simulink library "tqr"  (R2021b)
settings: Solver=VariableStepAuto  StartTime=0.0  StopTime=10.0  RelTol=1e-3
undefined symbols (not defined in the file or in its folder): ATQR_AltRDCActiveFEDUInc_X_pct, ATQR_AltRDCActiveFEDUInc_Y_enum, ATQR_AltRDCActiveFEDUTs_X_pct, ATQR_AltRDCActiveFEDUTs_Y_enum, ATQR_AltRDCActiveREDUInc_X_pct, ATQR_AltRDCActiveREDUInc_Y_enum, ATQR_AltRDCActiveREDUTs_X_pct, ATQR_AltRDCActiveREDUTs_Y_enum, ATQR_CreepFEDUTqIncSR_X_rpm, ATQR_CreepFEDUTqIncSR_Y_Nm, ATQR_CreepFEDUTs_X_rpm, ATQR_CreepFEDUTs_Y_Nm, ATQR_ECO2TqFrIncGain_X_Nm, ATQR_ECO2TqFrIncGain_Y_pct, ATQR_ECO2TqRrIncGain_X_Nm, ATQR_ECO2TqRrIncGain_Y_pct, ATQR_EcoTqFrIncGain_X_Nm, ATQR_EcoTqFrIncGain_Y_pct, ATQR_EcoTqRrIncGain_X_Nm, ATQR_EcoTqRrIncGain_Y_pct, ATQR_EL1FEDUTqDecSR_Y_Nm, ATQR_EL1FEDUTqIncSR_X_rpm, ATQR_EL1FEDUTqIncSR_Y_pct, ATQR_EL1FEDUTs_X_rpm, ATQR_EL1FEDUTs_Y_Nm, ATQR_EL1REDUTqDecSR_Y_Nm, ATQR_EL1REDUTs_Y_Nm, ATQR_FEDUEL1RegenTs_X_rpm, ATQR_FEDUTIPOutTs_X_rpm, ATQR_FrNegRateLimitIncN_X_rpm, ATQR_FrNegRateLimitIncN_Y_Nm, ATQR_FrPosRateLimitIncN_X_rpm, ATQR_FrPosRateLimitIncN_Y_Nm, ATQR_FShaftSpdTqLimCoe_X_rpm, ATQR_FTimerTqLimCoe_X_s, ATQR_FTqZeroTransUpBoundN_X_rpm, ATQR_NL1FEDUTqDecSR_Y_Nm, ATQR_NL1FEDUTqIncSR_X_rpm, ATQR_NL1FEDUTqIncSR_Y_pct, ATQR_NL1FEDUTs_X_rpm, ATQR_NL1FEDUTs_Y_Nm, ATQR_NL1REDUTqDecSR_Y_Nm, ATQR_NL1REDUTs_Y_Nm, ATQR_NL2TqFrIncGain_X_Nm, ATQR_NL2TqFrIncGain_Y_pct, ATQR_NL2TqRrIncGain_X_Nm, ATQR_NL2TqRrIncGain_Y_pct, ATQR_NormalTqFrIncGain_X_Nm, ATQR_NormalTqFrIncGain_Y_pct, ATQR_NormalTqRrIncGain_X_Nm, ATQR_NormalTqRrIncGain_Y_pct, ATQR_RrNegRateLimitIncN_X_rpm, ATQR_RrNegRateLimitIncN_Y_Nm, ATQR_RrPosRateLimitIncN_X_rpm, ATQR_RrPosRateLimitIncN_Y_Nm, ATQR_RShaftSpdTqLimCoe_X_rpm, ATQR_RTimerTqLimCoe_X_s, ATQR_SL1FEDUTqDecSR_Y_Nm, ATQR_SL1FEDUTqIncSR_X_rpm, ATQR_SL1FEDUTqIncSR_Y_pct ... (+344)
libraries: hcu_lib x23, simulink x17, $bdroot x3
(part 9 of 12)

== system tqr/TQR/Determine Torque Request/TorqueArbitrament/TorqueSmooth/Rear wheel rate limit determination/VTQR_ECOREDURateLimitInc_Nm ==
  VDHP_ActAPSPosn_pct : Inport
  VTQD_TqTargetShaftSpd_rpm : Inport  Port=2
  VTQD_RegenMode_enum : Inport  Port=3
  VTQR_REDUWhlTqReqSmoothDelay_Nm : Inport  Port=4
  Action Port : ActionPort
  Constant : Constant  Value=ENUM_REGENLEVEL_LV1
  Constant1 : Constant  Value=ENUM_REGENLEVEL_LV2
  Constant2 : Constant  Value=ENUM_REGENLEVEL_LV3
  Constant3 : Constant  Value=ENUM_REGENLEVEL_LV4
  Constant4 : Constant  Value=ENUM_REGENLEVEL_LV5
  Constant5 : Constant  Value=ENUM_REGENLEVEL_OPD
  Constant6 : Constant  Value=KTQR_EnEcoRrIncGain_enum
  Constant7 : Constant  Value=ONE_FLOAT
  Equal{,1..5} (6 alike) : RelationalOperator  Operator===  OutDataTypeStr=boolean  RndMeth=Simplest
  If : If  NumInputs=6  IfExpression=u1~= 0  ElseIfExpressions=u2 ~= 0, u3 ~= 0,u4 ~= 0,u5~=0,u6~=0
  Invalid : Subsystem  TreatAsAtomicUnit=on
  LV1 : Subsystem  TreatAsAtomicUnit=on
  LV2 : Subsystem  TreatAsAtomicUnit=on
  LV3 : Subsystem  TreatAsAtomicUnit=on
  LV4 : Subsystem  TreatAsAtomicUnit=on
  LV5 : Subsystem  TreatAsAtomicUnit=on
  MTQR_ECO2TqRrIncGain_Z_c : Lookup_n-D  BreakpointsForDimension1=ATQR_ECO2TqRrIncGain_Y_pct  BreakpointsForDimension2=ATQR_ECO2TqRrIncGain_X_Nm  Table=MTQR_ECO2TqRrIncGain_Z_c  ExtrapMethod=Clip  InternalRulePriority=Speed  RndMeth=Simplest  InputSameDT=on
      settings: InputPortMap=u0,u1
  MTQR_ECO3TqRrIncGain_Z_c : Lookup_n-D  BreakpointsForDimension1=ATQR_ECO2TqRrIncGain_Y_pct  BreakpointsForDimension2=ATQR_ECO2TqRrIncGain_X_Nm  Table=MTQR_ECO3TqRrIncGain_Z_c  ExtrapMethod=Clip  InternalRulePriority=Speed  RndMeth=Simplest  InputSameDT=on
      settings: InputPortMap=u0,u1
  MTQR_ECO4TqRrIncGain_Z_c : Lookup_n-D  BreakpointsForDimension1=ATQR_ECO2TqRrIncGain_Y_pct  BreakpointsForDimension2=ATQR_ECO2TqRrIncGain_X_Nm  Table=MTQR_ECO4TqRrIncGain_Z_c  ExtrapMethod=Clip  InternalRulePriority=Speed  RndMeth=Simplest  InputSameDT=on
      settings: InputPortMap=u0,u1
  MTQR_ECO5TqRrIncGain_Z_c : Lookup_n-D  BreakpointsForDimension1=ATQR_ECO2TqRrIncGain_Y_pct  BreakpointsForDimension2=ATQR_ECO2TqRrIncGain_X_Nm  Table=MTQR_ECO5TqRrIncGain_Z_c  ExtrapMethod=Clip  InternalRulePriority=Speed  RndMeth=Simplest  InputSameDT=on
      settings: InputPortMap=u0,u1
  MTQR_ECOOPDTqRrIncGain_Z_c : Lookup_n-D  BreakpointsForDimension1=ATQR_ECO2TqRrIncGain_Y_pct  BreakpointsForDimension2=ATQR_ECO2TqRrIncGain_X_Nm  Table=MTQR_ECOOPDTqRrIncGain_Z_c  ExtrapMethod=Clip  InternalRulePriority=Speed  RndMeth=Simplest  InputSameDT=on
      settings: InputPortMap=u0,u1
  MTQR_EcoTqRrIncGain_Z_c : Lookup_n-D  BreakpointsForDimension1=ATQR_EcoTqRrIncGain_Y_pct  BreakpointsForDimension2=ATQR_EcoTqRrIncGain_X_Nm  Table=MTQR_EcoTqRrIncGain_Z_c  ExtrapMethod=Clip  InternalRulePriority=Speed  RndMeth=Simplest  InputSameDT=on
      settings: InputPortMap=u0,u1
  Merge : Merge  Inputs=7
  OPD : Subsystem  TreatAsAtomicUnit=on
  Relational Operator : RelationalOperator  OutDataTypeStr=boolean  RndMeth=Simplest
  Switch : Switch  Criteria=u2 > Threshold
  VTQR_ECOREDURateLimitInc_Nm : Outport
  wires:
  [VDHP_ActAPSPosn_pct] -> MTQR_ECOOPDTqRrIncGain_Z_c/1
  [VTQR_REDUWhlTqReqSmoothDelay_Nm] -> MTQR_ECOOPDTqRrIncGain_Z_c/2
  [VDHP_ActAPSPosn_pct] -> MTQR_ECO5TqRrIncGain_Z_c/1
  [VTQR_REDUWhlTqReqSmoothDelay_Nm] -> MTQR_ECO5TqRrIncGain_Z_c/2
  [VTQR_REDUWhlTqReqSmoothDelay_Nm] -> MTQR_ECO4TqRrIncGain_Z_c/2
  [VDHP_ActAPSPosn_pct] -> MTQR_ECO4TqRrIncGain_Z_c/1
  [VTQR_REDUWhlTqReqSmoothDelay_Nm] -> MTQR_ECO3TqRrIncGain_Z_c/2
  [VDHP_ActAPSPosn_pct] -> MTQR_ECO3TqRrIncGain_Z_c/1
  [VTQR_REDUWhlTqReqSmoothDelay_Nm] -> MTQR_ECO2TqRrIncGain_Z_c/2
  [VDHP_ActAPSPosn_pct] -> MTQR_ECO2TqRrIncGain_Z_c/1
  If/7 -> Invalid/Action
  If/6 -> OPD/Action
  [VTQR_ECOOPDTqRrIncGain_c] -> OPD/4(VTQR_ECOOPDTqRrIncGain_c)
  If/5 -> LV5/Action
  [VTQR_ECO5TqRrIncGain_c] -> LV5/4(VTQR_ECO5TqRrIncGain_c)
  If/4 -> LV4/Action
  [VTQR_ECO4TqRrIncGain_c] -> LV4/4(VTQR_ECO4TqRrIncGain_c)
  If/3 -> LV3/Action
  [VTQR_ECO3TqRrIncGain_c] -> LV3/4(VTQR_ECO3TqRrIncGain_c)
  If/2 -> LV2/Action
  [VTQR_ECO2TqRrIncGain_c] -> LV2/4(VTQR_ECO2TqRrIncGain_c)
  If/1 -> LV1/Action
  MTQR_ECO5TqRrIncGain_Z_c/1 -> [VTQR_ECO5TqRrIncGain_c]  "VTQR_ECO5TqRrIncGain_c"
  MTQR_ECO2TqRrIncGain_Z_c/1 -> [VTQR_ECO2TqRrIncGain_c]  "VTQR_ECO2TqRrIncGain_c"
  MTQR_ECOOPDTqRrIncGain_Z_c/1 -> [VTQR_ECOOPDTqRrIncGain_c]  "VTQR_ECOOPDTqRrIncGain_c"
  MTQR_ECO3TqRrIncGain_Z_c/1 -> [VTQR_ECO3TqRrIncGain_c]  "VTQR_ECO3TqRrIncGain_c"
  MTQR_ECO4TqRrIncGain_Z_c/1 -> [VTQR_ECO4TqRrIncGain_c]  "VTQR_ECO4TqRrIncGain_c"
  Switch/1 -> [VTQR_EcoTqRrIncGain_c]  "VTQR_EcoTqRrIncGain_c"
  MTQR_EcoTqRrIncGain_Z_c/1 -> Switch/1
  [VTQD_RegenMode_enum] -> Relational Operator/1
  Constant6/1 -> Relational Operator/2
  Constant7/1 -> Switch/3
  Relational Operator/1 -> Switch/2
  [VTQR_EcoTqRrIncGain_c] -> OPD/3(VTQR_EcoTqRrIncGain_c)
  [VTQR_EcoTqRrIncGain_c] -> LV5/3(VTQR_EcoTqRrIncGain_c)
  [VTQR_EcoTqRrIncGain_c] -> LV4/3(VTQR_EcoTqRrIncGain_c)
  [VTQR_EcoTqRrIncGain_c] -> LV3/3(VTQR_EcoTqRrIncGain_c)
  [VTQR_EcoTqRrIncGain_c] -> LV2/3(VTQR_EcoTqRrIncGain_c)
  [VTQR_EcoTqRrIncGain_c] -> LV1/3(VTQR_EcoTqRrIncGain_c)
  VTQR_REDUWhlTqReqSmoothDelay_Nm/1 -> [VTQR_REDUWhlTqReqSmoothDelay_Nm]
  [VDHP_ActAPSPosn_pct] -> MTQR_EcoTqRrIncGain_Z_c/1
  [VTQR_REDUWhlTqReqSmoothDelay_Nm] -> MTQR_EcoTqRrIncGain_Z_c/2
  Invalid/1(VTQR_EL1REDUTqIncSR_Nm) -> Merge/7
  [VTQD_TqTargetShaftSpd_rpm] -> Invalid/2(VTQD_TqTargetShaftSpd_rpm)
  [VDHP_ActAPSPosn_pct] -> Invalid/1(VDHP_ActAPSPosn_pct)
  VTQD_RegenMode_enum/1 -> [VTQD_RegenMode_enum]
  VTQD_TqTargetShaftSpd_rpm/1 -> [VTQD_TqTargetShaftSpd_rpm]
  VDHP_ActAPSPosn_pct/1 -> [VDHP_ActAPSPosn_pct]
  Merge/1 -> VTQR_ECOREDURateLimitInc_Nm/1  "VTQR_ECOREDURateLimitInc_Nm"
  Constant2/1 -> Equal2/2
  [VDHP_ActAPSPosn_pct] -> LV1/1(VDHP_ActAPSPosn_pct)
  [VTQD_TqTargetShaftSpd_rpm] -> LV3/2(VTQD_TqTargetShaftSpd_rpm)
  LV4/1(VTQR_EL4REDUTqIncSR_Nm) -> Merge/4
  Equal3/1 -> If/4
  [VTQD_RegenMode_enum] -> Equal1/1
  LV5/1(VTQR_EL5REDUTqIncSR_Nm) -> Merge/5
  LV3/1(VTQR_EL3REDUTqIncSR_Nm) -> Merge/3
  [VTQD_RegenMode_enum] -> Equal3/1
  Equal1/1 -> If/2
  Equal4/1 -> If/5
  [VTQD_RegenMode_enum] -> Equal/1
  LV1/1(VTQR_EL1REDUTqIncSR_Nm) -> Merge/1
  Constant1/1 -> Equal1/2
  Equal/1 -> If/1
  [VTQD_TqTargetShaftSpd_rpm] -> LV5/2(VTQD_TqTargetShaftSpd_rpm)
  [VDHP_ActAPSPosn_pct] -> LV4/1(VDHP_ActAPSPosn_pct)
  Constant5/1 -> Equal5/2
  [VDHP_ActAPSPosn_pct] -> LV3/1(VDHP_ActAPSPosn_pct)
  [VTQD_TqTargetShaftSpd_rpm] -> LV4/2(VTQD_TqTargetShaftSpd_rpm)
  [VTQD_TqTargetShaftSpd_rpm] -> OPD/2(VTQD_TqTargetShaftSpd_rpm)
  [VDHP_ActAPSPosn_pct] -> LV5/1(VDHP_ActAPSPosn_pct)
  [VTQD_TqTargetShaftSpd_rpm] -> LV1/2(VTQD_TqTargetShaftSpd_rpm)
  [VTQD_RegenMode_enum] -> Equal2/1
  [VDHP_ActAPSPosn_pct] -> OPD/1(VDHP_ActAPSPosn_pct)
  [VTQD_RegenMode_enum] -> Equal5/1
  LV2/1(VTQR_EL2REDUTqIncSR_Nm) -> Merge/2
  [VDHP_ActAPSPosn_pct] -> LV2/1(VDHP_ActAPSPosn_pct)
  [VTQD_RegenMode_enum] -> Equal4/1
  OPD/1(VTQR_EOPDREDUTqIncSR_Nm) -> Merge/6
  Equal5/1 -> If/6
  Constant/1 -> Equal/2
  Constant4/1 -> Equal4/2
  Equal2/1 -> If/3
  Constant3/1 -> Equal3/2
  [VTQD_TqTargetShaftSpd_rpm] -> LV2/2(VTQD_TqTargetShaftSpd_rpm)

== system tqr/TQR/Determine Torque Request/TorqueArbitrament/TorqueSmooth/Rear wheel rate limit determination/VTQR_ESCAPEREDURateLimitDec_Nm ==
  VTQR_REDUWhlTqReqSmoothDelay_Nm : Inport
  VTQD_RrShaftSpd_rpm : Inport  Port=2
  Action Port : ActionPort
  MTQR_ESCAPEREDUTqDecSR_Z_Nm : Lookup_n-D  BreakpointsForDimension1=ATQR_NL1REDUTqDecSR_Y_Nm  BreakpointsForDimension2=ATQR_NL1FEDUTqIncSR_X_rpm  Table=MTQR_ESCAPEREDUTqDecSR_Z_Nm  InternalRulePriority=Speed  RndMeth=Simplest  InputSameDT=on
      settings: InputPortMap=u0,u1
  VTQR_ESCAPEREDURateLimitDec_Nm : Outport
  wires:
  MTQR_ESCAPEREDUTqDecSR_Z_Nm/1 -> VTQR_ESCAPEREDURateLimitDec_Nm/1
  VTQR_REDUWhlTqReqSmoothDelay_Nm/1 -> MTQR_ESCAPEREDUTqDecSR_Z_Nm/1
  VTQD_RrShaftSpd_rpm/1 -> MTQR_ESCAPEREDUTqDecSR_Z_Nm/2

== system tqr/TQR/Determine Torque Request/TorqueArbitrament/TorqueSmooth/Rear wheel rate limit determination/VTQR_ESCAPEREDURateLimitInc_Nm ==
  VDHP_ActAPSPosn_pct : Inport
  VTQD_RrShaftSpd_rpm : Inport  Port=2
  Action Port : ActionPort
  MTQR_ESCAPEREDUTqIncSR_Z_Nm : Lookup_n-D  BreakpointsForDimension1=ATQR_NL1FEDUTqIncSR_Y_pct  BreakpointsForDimension2=ATQR_NL1FEDUTqIncSR_X_rpm  Table=MTQR_ESCAPEREDUTqIncSR_Z_Nm  InternalRulePriority=Speed  RndMeth=Simplest  InputSameDT=on
      settings: InputPortMap=u0,u1
  VTQR_ESCAPEREDURateLimitInc_Nm : Outport
  wires:
  VDHP_ActAPSPosn_pct/1 -> MTQR_ESCAPEREDUTqIncSR_Z_Nm/1
  VTQD_RrShaftSpd_rpm/1 -> MTQR_ESCAPEREDUTqIncSR_Z_Nm/2
  MTQR_ESCAPEREDUTqIncSR_Z_Nm/1 -> VTQR_ESCAPEREDURateLimitInc_Nm/1

== system tqr/TQR/Determine Torque Request/TorqueArbitrament/TorqueSmooth/Rear wheel rate limit determination/VTQR_LHMREDURateLimitDec_Nm ==
  VTQR_REDUWhlTqReqSmooth_Nm : Inport
  VTQD_TqTargetShaftSpd_rpm : Inport  Port=2
  Action Port : ActionPort
  MTQR_LHMREDUTqDecSR_Z_Nm : Lookup_n-D  BreakpointsForDimension1=ATQR_NL1REDUTqDecSR_Y_Nm  BreakpointsForDimension2=ATQR_NL1FEDUTqIncSR_X_rpm  Table=MTQR_LHMREDUTqDecSR_Z_Nm  ExtrapMethod=Clip  InternalRulePriority=Speed  RndMeth=Simplest  InputSameDT=on
      settings: InputPortMap=u0,u1
  VTQR_LHMREDURateLimitDec_Nm : Outport
  wires:
  MTQR_LHMREDUTqDecSR_Z_Nm/1 -> VTQR_LHMREDURateLimitDec_Nm/1  "VTQR_LHMREDURateLimitDec_Nm"
  VTQD_TqTargetShaftSpd_rpm/1 -> MTQR_LHMREDUTqDecSR_Z_Nm/2
  VTQR_REDUWhlTqReqSmooth_Nm/1 -> MTQR_LHMREDUTqDecSR_Z_Nm/1

== system tqr/TQR/Determine Torque Request/TorqueArbitrament/TorqueSmooth/Rear wheel rate limit determination/VTQR_LHMREDURateLimitInc_Nm ==
  VDHP_ActAPSPosn_pct : Inport
  VTQD_TqTargetShaftSpd_rpm : Inport  Port=2
  Action Port : ActionPort
  MTQR_LHMREDUTqIncSR_Z_Nm : Lookup_n-D  BreakpointsForDimension1=ATQR_NL1FEDUTqIncSR_Y_pct  BreakpointsForDimension2=ATQR_NL1FEDUTqIncSR_X_rpm  Table=MTQR_LHMREDUTqIncSR_Z_Nm  ExtrapMethod=Clip  InternalRulePriority=Speed  RndMeth=Simplest  InputSameDT=on
      settings: InputPortMap=u0,u1
  VTQR_LHMREDURateLimitInc_Nm : Outport
  wires:
  MTQR_LHMREDUTqIncSR_Z_Nm/1 -> VTQR_LHMREDURateLimitInc_Nm/1  "VTQR_LHMREDURateLimitInc_Nm"
  VTQD_TqTargetShaftSpd_rpm/1 -> MTQR_LHMREDUTqIncSR_Z_Nm/2
  VDHP_ActAPSPosn_pct/1 -> MTQR_LHMREDUTqIncSR_Z_Nm/1

== system tqr/TQR/Determine Torque Request/TorqueArbitrament/TorqueSmooth/Rear wheel rate limit determination/VTQR_NORMALREDURateLimitDec_Nm ==
  VTQR_REDUWhlTqReqSmoothDelay_Nm : Inport
  VTQD_TqTargetShaftSpd_rpm : Inport  Port=2
  VTQD_RegenMode_enum : Inport  Port=3
  Action Port : ActionPort
  Constant : Constant  Value=ENUM_REGENLEVEL_LV1
  Constant1 : Constant  Value=ENUM_REGENLEVEL_LV2
  Constant2 : Constant  Value=ENUM_REGENLEVEL_LV3
  Constant3 : Constant  Value=ENUM_REGENLEVEL_LV4
  Constant4 : Constant  Value=ENUM_REGENLEVEL_LV5
  Constant5 : Constant  Value=ENUM_REGENLEVEL_OPD
  Equal{,1..5} (6 alike) : RelationalOperator  Operator===  OutDataTypeStr=boolean  RndMeth=Simplest
  If : If  NumInputs=6  IfExpression=u1~= 0  ElseIfExpressions=u2 ~= 0, u3 ~= 0,u4 ~= 0,u5~=0,u6~=0
  Invalid : Subsystem  TreatAsAtomicUnit=on
  LV1 : Subsystem  TreatAsAtomicUnit=on
  LV2 : Subsystem  AncestorBlock=tqr/TQR/Determine Torque Request/TorqueArbitrament/TorqueSmooth/Front First order filter input tau map and determination/VTQR_ECOFEDUTs_c/LV2  TreatAsAtomicUnit=on
  LV3 : Subsystem  AncestorBlock=tqr/TQR/Determine Torque Request/TorqueArbitrament/TorqueSmooth/Front First order filter input tau map and determination/VTQR_ECOFEDUTs_c/LV3  TreatAsAtomicUnit=on
  LV4 : Subsystem  AncestorBlock=tqr/TQR/Determine Torque Request/TorqueArbitrament/TorqueSmooth/Front First order filter input tau map and determination/VTQR_ECOFEDUTs_c/LV4  TreatAsAtomicUnit=on
  LV5 : Subsystem  AncestorBlock=tqr/TQR/Determine Torque Request/TorqueArbitrament/TorqueSmooth/Front First order filter input tau map and determination/VTQR_ECOFEDUTs_c/LV5  TreatAsAtomicUnit=on
  Merge : Merge  Inputs=7
  OPD : Subsystem  AncestorBlock=tqr/TQR/Determine Torque Request/TorqueArbitrament/TorqueSmooth/Front First order filter input tau map and determination/VTQR_ECOFEDUTs_c/OPD  TreatAsAtomicUnit=on
  VTQR_NORMALREDURateLimitDec_Nm : Outport
  wires:
  Invalid/1(VTQR_NL1REDUTqDecSR_Nm) -> Merge/7
  If/7 -> Invalid/Action
  [VTQD_TqTargetShaftSpd_rpm] -> Invalid/2(VTQD_TqTargetShaftSpd_rpm)
  [VTQR_REDUWhlTqReqSmoothDelay_Nm] -> Invalid/1(VTQR_REDUWhlTqReqSmoothDelay_Nm)
  If/6 -> OPD/Action
  If/5 -> LV5/Action
  If/4 -> LV4/Action
  If/3 -> LV3/Action
  If/2 -> LV2/Action
  If/1 -> LV1/Action
  VTQD_RegenMode_enum/1 -> [VTQD_RegenMode_enum]
  VTQD_TqTargetShaftSpd_rpm/1 -> [VTQD_TqTargetShaftSpd_rpm]
  VTQR_REDUWhlTqReqSmoothDelay_Nm/1 -> [VTQR_REDUWhlTqReqSmoothDelay_Nm]
  Merge/1 -> VTQR_NORMALREDURateLimitDec_Nm/1  "VTQR_NORMALREDURateLimitDec_Nm"
  Constant2/1 -> Equal2/2
  [VTQR_REDUWhlTqReqSmoothDelay_Nm] -> LV1/1(VTQR_REDUWhlTqReqSmoothDelay_Nm)
  [VTQD_TqTargetShaftSpd_rpm] -> LV3/2(VTQD_TqTargetShaftSpd_rpm)
  LV4/1(VTQR_NL4REDUTqDecSR_Nm) -> Merge/4
  Equal3/1 -> If/4
  [VTQD_RegenMode_enum] -> Equal1/1
  LV5/1(VTQR_NL5REDUTqDecSR_Nm) -> Merge/5
  LV3/1(VTQR_NL3REDUTqDecSR_Nm) -> Merge/3
  [VTQD_RegenMode_enum] -> Equal3/1
  Equal1/1 -> If/2
  Equal4/1 -> If/5
  [VTQD_RegenMode_enum] -> Equal/1
  LV1/1(VTQR_NL1REDUTqDecSR_Nm) -> Merge/1
  Constant1/1 -> Equal1/2
  Equal/1 -> If/1
  [VTQD_TqTargetShaftSpd_rpm] -> LV5/2(VTQD_TqTargetShaftSpd_rpm)
  [VTQR_REDUWhlTqReqSmoothDelay_Nm] -> LV4/1(VTQR_REDUWhlTqReqSmoothDelay_Nm)
  Constant5/1 -> Equal5/2
  [VTQR_REDUWhlTqReqSmoothDelay_Nm] -> LV3/1(VTQR_REDUWhlTqReqSmoothDelay_Nm)
  [VTQD_TqTargetShaftSpd_rpm] -> LV4/2(VTQD_TqTargetShaftSpd_rpm)
  [VTQD_TqTargetShaftSpd_rpm] -> OPD/2(VTQD_TqTargetShaftSpd_rpm)
  [VTQR_REDUWhlTqReqSmoothDelay_Nm] -> LV5/1(VTQR_REDUWhlTqReqSmoothDelay_Nm)
  [VTQD_TqTargetShaftSpd_rpm] -> LV1/2(VTQD_TqTargetShaftSpd_rpm)
  [VTQD_RegenMode_enum] -> Equal2/1
  [VTQR_REDUWhlTqReqSmoothDelay_Nm] -> OPD/1(VTQR_REDUWhlTqReqSmoothDelay_Nm)
  [VTQD_RegenMode_enum] -> Equal5/1
  LV2/1(VTQR_NL2REDUTqDecSR_Nm) -> Merge/2
  [VTQR_REDUWhlTqReqSmoothDelay_Nm] -> LV2/1(VTQR_REDUWhlTqReqSmoothDelay_Nm)
  [VTQD_RegenMode_enum] -> Equal4/1
  OPD/1(VTQR_NOPDREDUTqDecSR_Nm) -> Merge/6
  Equal5/1 -> If/6
  Constant/1 -> Equal/2
  Constant4/1 -> Equal4/2
  Equal2/1 -> If/3
  Constant3/1 -> Equal3/2
  [VTQD_TqTargetShaftSpd_rpm] -> LV2/2(VTQD_TqTargetShaftSpd_rpm)

== system tqr/TQR/Determine Torque Request/TorqueArbitrament/TorqueSmooth/Rear wheel rate limit determination/VTQR_NORMALREDURateLimitInc_Nm ==
  VDHP_ActAPSPosn_pct : Inport
  VTQD_TqTargetShaftSpd_rpm : Inport  Port=2
  VTQD_RegenMode_enum : Inport  Port=3
  VTQR_REDUWhlTqReqSmoothDelay_Nm : Inport  Port=4
  Action Port : ActionPort
  Constant : Constant  Value=ENUM_REGENLEVEL_LV1
  Constant1 : Constant  Value=ENUM_REGENLEVEL_LV2
  Constant2 : Constant  Value=ENUM_REGENLEVEL_LV3
  Constant3 : Constant  Value=ENUM_REGENLEVEL_LV4
  Constant4 : Constant  Value=ENUM_REGENLEVEL_LV5
  Constant5 : Constant  Value=ENUM_REGENLEVEL_OPD
  Constant6 : Constant  Value=KTQR_EnNormalRrIncGain_enum
  Constant7 : Constant  Value=ONE_FLOAT
  Equal{,1..5} (6 alike) : RelationalOperator  Operator===  OutDataTypeStr=boolean  RndMeth=Simplest
  If : If  NumInputs=6  IfExpression=u1~= 0  ElseIfExpressions=u2 ~= 0, u3 ~= 0,u4 ~= 0,u5~=0,u6~=0
  Invalid : Subsystem  TreatAsAtomicUnit=on
  LV1 : Subsystem  TreatAsAtomicUnit=on
  LV2 : Subsystem  TreatAsAtomicUnit=on
  LV3 : Subsystem  TreatAsAtomicUnit=on
  LV4 : Subsystem  TreatAsAtomicUnit=on
  LV5 : Subsystem  TreatAsAtomicUnit=on
  MTQR_NL2TqRrIncGain_Z_c : Lookup_n-D  BreakpointsForDimension1=ATQR_NL2TqRrIncGain_Y_pct  BreakpointsForDimension2=ATQR_NL2TqRrIncGain_X_Nm  Table=MTQR_NL2TqRrIncGain_Z_c  ExtrapMethod=Clip  InternalRulePriority=Speed  RndMeth=Simplest  InputSameDT=on
      settings: InputPortMap=u0,u1
  MTQR_NL3TqRrIncGain_Z_c : Lookup_n-D  BreakpointsForDimension1=ATQR_NL2TqRrIncGain_Y_pct  BreakpointsForDimension2=ATQR_NL2TqRrIncGain_X_Nm  Table=MTQR_NL3TqRrIncGain_Z_c  ExtrapMethod=Clip  InternalRulePriority=Speed  RndMeth=Simplest  InputSameDT=on
      settings: InputPortMap=u0,u1
  MTQR_NL4TqRrIncGain_Z_c : Lookup_n-D  BreakpointsForDimension1=ATQR_NL2TqRrIncGain_Y_pct  BreakpointsForDimension2=ATQR_NL2TqRrIncGain_X_Nm  Table=MTQR_NL4TqRrIncGain_Z_c  ExtrapMethod=Clip  InternalRulePriority=Speed  RndMeth=Simplest  InputSameDT=on
      settings: InputPortMap=u0,u1
  MTQR_NL5TqRrIncGain_Z_c : Lookup_n-D  BreakpointsForDimension1=ATQR_NL2TqRrIncGain_Y_pct  BreakpointsForDimension2=ATQR_NL2TqRrIncGain_X_Nm  Table=MTQR_NL5TqRrIncGain_Z_c  ExtrapMethod=Clip  InternalRulePriority=Speed  RndMeth=Simplest  InputSameDT=on
      settings: InputPortMap=u0,u1
  MTQR_NLOPDTqRrIncGain_Z_c : Lookup_n-D  BreakpointsForDimension1=ATQR_NL2TqRrIncGain_Y_pct  BreakpointsForDimension2=ATQR_NL2TqRrIncGain_X_Nm  Table=MTQR_NLOPDTqRrIncGain_Z_c  ExtrapMethod=Clip  InternalRulePriority=Speed  RndMeth=Simplest  InputSameDT=on
      settings: InputPortMap=u0,u1
  MTQR_NormalTqRrIncGain_Z_c : Lookup_n-D  BreakpointsForDimension1=ATQR_NormalTqRrIncGain_Y_pct  BreakpointsForDimension2=ATQR_NormalTqRrIncGain_X_Nm  Table=MTQR_NormalTqRrIncGain_Z_c  ExtrapMethod=Clip  InternalRulePriority=Speed  RndMeth=Simplest  InputSameDT=on
      settings: InputPortMap=u0,u1
  Merge : Merge  Inputs=7
  OPD : Subsystem  TreatAsAtomicUnit=on
  Relational Operator : RelationalOperator  OutDataTypeStr=boolean  RndMeth=Simplest
  Switch : Switch  Criteria=u2 > Threshold
  VTQR_NORMALREDURateLimitInc_Nm : Outport
  wires:
  [VTQR_REDUWhlTqReqSmoothDelay_Nm] -> MTQR_NLOPDTqRrIncGain_Z_c/2
  [VTQR_REDUWhlTqReqSmoothDelay_Nm] -> MTQR_NL5TqRrIncGain_Z_c/2
  [VTQR_REDUWhlTqReqSmoothDelay_Nm] -> MTQR_NL4TqRrIncGain_Z_c/2
  [VTQR_REDUWhlTqReqSmoothDelay_Nm] -> MTQR_NL3TqRrIncGain_Z_c/2
  [VTQR_REDUWhlTqReqSmoothDelay_Nm] -> MTQR_NL2TqRrIncGain_Z_c/2
  [VTQR_NLOPDTqRrIncGain_c] -> OPD/4(VTQR_NLOPDTqRrIncGain_c)
  If/7 -> Invalid/Action
  [VTQR_NL5TqRrIncGain_c] -> LV5/4(VTQR_NL5TqRrIncGain_c)
  [VTQR_NL4TqRrIncGain_c] -> LV4/4(VTQR_NL4TqRrIncGain_c)
  [VTQR_NL3TqRrIncGain_c] -> LV3/4(VTQR_NL3TqRrIncGain_c)
  If/1 -> LV1/Action
  If/2 -> LV2/Action
  If/3 -> LV3/Action
  If/4 -> LV4/Action
  If/5 -> LV5/Action
  If/6 -> OPD/Action
  [VTQR_NL2TqRrIncGain_c] -> LV2/4(VTQR_NL2TqRrIncGain_c)
  [VDHP_ActAPSPosn_pct] -> MTQR_NL4TqRrIncGain_Z_c/1
  [VDHP_ActAPSPosn_pct] -> MTQR_NL2TqRrIncGain_Z_c/1
  MTQR_NL5TqRrIncGain_Z_c/1 -> [VTQR_NL5TqRrIncGain_c]  "VTQR_NL5TqRrIncGain_c"
  [VDHP_ActAPSPosn_pct] -> MTQR_NL5TqRrIncGain_Z_c/1
  [VDHP_ActAPSPosn_pct] -> MTQR_NLOPDTqRrIncGain_Z_c/1
  MTQR_NLOPDTqRrIncGain_Z_c/1 -> [VTQR_NLOPDTqRrIncGain_c]  "VTQR_NLOPDTqRrIncGain_c"
  MTQR_NL2TqRrIncGain_Z_c/1 -> [VTQR_NL2TqRrIncGain_c]  "VTQR_NL2TqRrIncGain_c"
  MTQR_NL3TqRrIncGain_Z_c/1 -> [VTQR_NL3TqRrIncGain_c]  "VTQR_NL3TqRrIncGain_c"
  [VDHP_ActAPSPosn_pct] -> MTQR_NL3TqRrIncGain_Z_c/1
  MTQR_NL4TqRrIncGain_Z_c/1 -> [VTQR_NL4TqRrIncGain_c]  "VTQR_NL4TqRrIncGain_c"
  Constant7/1 -> Switch/3
  Constant6/1 -> Relational Operator/2
  [VTQD_RegenMode_enum] -> Relational Operator/1
  Relational Operator/1 -> Switch/2
  Switch/1 -> [VTQR_NormalTqRrIncGain_c]  "VTQR_NormalTqRrIncGain_c"
  MTQR_NormalTqRrIncGain_Z_c/1 -> Switch/1
  [VTQR_NormalTqRrIncGain_c] -> LV1/3(VTQR_NormalTqRrIncGain_c)
  [VTQR_NormalTqRrIncGain_c] -> LV4/3(VTQR_NormalTqRrIncGain_c)
  [VTQR_NormalTqRrIncGain_c] -> LV5/3(VTQR_NormalTqRrIncGain_c)
  [VTQR_NormalTqRrIncGain_c] -> OPD/3(VTQR_NormalTqRrIncGain_c)
  [VTQR_NormalTqRrIncGain_c] -> LV3/3(VTQR_NormalTqRrIncGain_c)
  [VTQR_NormalTqRrIncGain_c] -> LV2/3(VTQR_NormalTqRrIncGain_c)
  [VTQR_REDUWhlTqReqSmoothDelay_Nm] -> MTQR_NormalTqRrIncGain_Z_c/2
  VTQR_REDUWhlTqReqSmoothDelay_Nm/1 -> [VTQR_REDUWhlTqReqSmoothDelay_Nm]
  [VDHP_ActAPSPosn_pct] -> MTQR_NormalTqRrIncGain_Z_c/1
  Invalid/1(VTQR_NL1REDUTqIncSR_Nm) -> Merge/7
  [VTQD_TqTargetShaftSpd_rpm] -> Invalid/2(VTQD_TqTargetShaftSpd_rpm)
  [VDHP_ActAPSPosn_pct] -> Invalid/1(VDHP_ActAPSPosn_pct)
  VTQD_RegenMode_enum/1 -> [VTQD_RegenMode_enum]
  [VTQD_RegenMode_enum] -> Equal4/1
  [VDHP_ActAPSPosn_pct] -> OPD/1(VDHP_ActAPSPosn_pct)
  Equal1/1 -> If/2
  [VDHP_ActAPSPosn_pct] -> LV1/1(VDHP_ActAPSPosn_pct)
  Equal5/1 -> If/6
  LV2/1(VTQR_NL2REDUTqIncSR_Nm) -> Merge/2
  [VTQD_TqTargetShaftSpd_rpm] -> LV5/2(VTQD_TqTargetShaftSpd_rpm)
  Equal3/1 -> If/4
  [VTQD_TqTargetShaftSpd_rpm] -> LV1/2(VTQD_TqTargetShaftSpd_rpm)
  Constant2/1 -> Equal2/2
  Equal2/1 -> If/3
  [VTQD_RegenMode_enum] -> Equal5/1
  [VTQD_TqTargetShaftSpd_rpm] -> LV2/2(VTQD_TqTargetShaftSpd_rpm)
  Constant4/1 -> Equal4/2
  OPD/1(VTQR_NOPDREDUTqIncSR_Nm) -> Merge/6
  [VDHP_ActAPSPosn_pct] -> LV3/1(VDHP_ActAPSPosn_pct)
  [VTQD_RegenMode_enum] -> Equal3/1
  Constant/1 -> Equal/2
  [VTQD_TqTargetShaftSpd_rpm] -> OPD/2(VTQD_TqTargetShaftSpd_rpm)
  Constant3/1 -> Equal3/2
  [VDHP_ActAPSPosn_pct] -> LV2/1(VDHP_ActAPSPosn_pct)
  [VDHP_ActAPSPosn_pct] -> LV5/1(VDHP_ActAPSPosn_pct)
  [VTQD_TqTargetShaftSpd_rpm] -> LV4/2(VTQD_TqTargetShaftSpd_rpm)
  [VTQD_RegenMode_enum] -> Equal2/1
  [VDHP_ActAPSPosn_pct] -> LV4/1(VDHP_ActAPSPosn_pct)
  Equal/1 -> If/1
  LV5/1(VTQR_NL5REDUTqIncSR_Nm) -> Merge/5
  Constant5/1 -> Equal5/2
  Equal4/1 -> If/5
  Constant1/1 -> Equal1/2
  [VTQD_RegenMode_enum] -> Equal/1
  LV1/1(VTQR_NL1REDUTqIncSR_Nm) -> Merge/1
  [VTQD_RegenMode_enum] -> Equal1/1
  LV4/1(VTQR_NL4REDUTqIncSR_Nm) -> Merge/4
  LV3/1(VTQR_NL3REDUTqIncSR_Nm) -> Merge/3
  [VTQD_TqTargetShaftSpd_rpm] -> LV3/2(VTQD_TqTargetShaftSpd_rpm)
  VTQD_TqTargetShaftSpd_rpm/1 -> [VTQD_TqTargetShaftSpd_rpm]
  Merge/1 -> VTQR_NORMALREDURateLimitInc_Nm/1  "VTQR_NORMALREDURateLimitInc_Nm"
  VDHP_ActAPSPosn_pct/1 -> [VDHP_ActAPSPosn_pct]

== system tqr/TQR/Determine Torque Request/TorqueArbitrament/TorqueSmooth/Rear wheel rate limit determination/VTQR_SNOWREDURateLimitDec_Nm ==
  VTQR_REDUWhlTqReqSmoothDelay_Nm : Inport
  VTQD_TqTargetShaftSpd_rpm : Inport  Port=2
  Action Port : ActionPort
  MTQR_SNOWREDUTqDecSR_Z_Nm : Lookup_n-D  BreakpointsForDimension1=ATQR_NL1REDUTqDecSR_Y_Nm  BreakpointsForDimension2=ATQR_NL1FEDUTqIncSR_X_rpm  Table=MTQR_SNOWREDUTqDecSR_Z_Nm  InternalRulePriority=Speed  RndMeth=Simplest  InputSameDT=on
      settings: InputPortMap=u0,u1
  VTQR_SNOWREDURateLimitDec_Nm : Outport
  wires:
  VTQD_TqTargetShaftSpd_rpm/1 -> MTQR_SNOWREDUTqDecSR_Z_Nm/2
  VTQR_REDUWhlTqReqSmoothDelay_Nm/1 -> MTQR_SNOWREDUTqDecSR_Z_Nm/1
  MTQR_SNOWREDUTqDecSR_Z_Nm/1 -> VTQR_SNOWREDURateLimitDec_Nm/1

== system tqr/TQR/Determine Torque Request/TorqueArbitrament/TorqueSmooth/Rear wheel rate limit determination/VTQR_SNOWREDURateLimitInc_Nm ==
  VDHP_ActAPSPosn_pct : Inport
  VTQD_TqTargetShaftSpd_rpm : Inport  Port=2
  Action Port : ActionPort
  MTQR_SNOWREDUTqIncSR_Z_Nm : Lookup_n-D  BreakpointsForDimension1=ATQR_NL1FEDUTqIncSR_Y_pct  BreakpointsForDimension2=ATQR_NL1FEDUTqIncSR_X_rpm  Table=MTQR_SNOWREDUTqIncSR_Z_Nm  InternalRulePriority=Speed  RndMeth=Simplest  InputSameDT=on
      settings: InputPortMap=u0,u1
  VTQR_SNOWREDURateLimitInc_Nm : Outport
  wires:
  MTQR_SNOWREDUTqIncSR_Z_Nm/1 -> VTQR_SNOWREDURateLimitInc_Nm/1
  VTQD_TqTargetShaftSpd_rpm/1 -> MTQR_SNOWREDUTqIncSR_Z_Nm/2
  VDHP_ActAPSPosn_pct/1 -> MTQR_SNOWREDUTqIncSR_Z_Nm/1

== system tqr/TQR/Determine Torque Request/TorqueArbitrament/TorqueSmooth/Rear wheel rate limit determination/VTQR_SPORTREDURateLimitDec_Nm ==
  VTQR_REDUWhlTqReqSmoothDelay_Nm : Inport
  VTQD_TqTargetShaftSpd_rpm : Inport  Port=2
  VTQD_RegenMode_enum : Inport  Port=3
  Action Port : ActionPort
  Constant : Constant  Value=ENUM_REGENLEVEL_LV1
  Constant1 : Constant  Value=ENUM_REGENLEVEL_LV2
  Constant2 : Constant  Value=ENUM_REGENLEVEL_LV3
  Constant3 : Constant  Value=ENUM_REGENLEVEL_LV4
  Constant4 : Constant  Value=ENUM_REGENLEVEL_LV5
  Constant5 : Constant  Value=ENUM_REGENLEVEL_OPD
  Equal{,1..5} (6 alike) : RelationalOperator  Operator===  OutDataTypeStr=boolean  RndMeth=Simplest
  If : If  NumInputs=6  IfExpression=u1~= 0  ElseIfExpressions=u2 ~= 0, u3 ~= 0,u4 ~= 0,u5~=0,u6~=0
  Invalid : Subsystem  TreatAsAtomicUnit=on
  LV1 : Subsystem  TreatAsAtomicUnit=on
  LV2 : Subsystem  AncestorBlock=tqr/TQR/Determine Torque Request/TorqueArbitrament/TorqueSmooth/Front First order filter input tau map and determination/VTQR_ECOFEDUTs_c/LV2  TreatAsAtomicUnit=on
  LV3 : Subsystem  AncestorBlock=tqr/TQR/Determine Torque Request/TorqueArbitrament/TorqueSmooth/Front First order filter input tau map and determination/VTQR_ECOFEDUTs_c/LV3  TreatAsAtomicUnit=on
  LV4 : Subsystem  AncestorBlock=tqr/TQR/Determine Torque Request/TorqueArbitrament/TorqueSmooth/Front First order filter input tau map and determination/VTQR_ECOFEDUTs_c/LV4  TreatAsAtomicUnit=on
  LV5 : Subsystem  AncestorBlock=tqr/TQR/Determine Torque Request/TorqueArbitrament/TorqueSmooth/Front First order filter input tau map and determination/VTQR_ECOFEDUTs_c/LV5  TreatAsAtomicUnit=on
  Merge : Merge  Inputs=7
  OPD : Subsystem  AncestorBlock=tqr/TQR/Determine Torque Request/TorqueArbitrament/TorqueSmooth/Front First order filter input tau map and determination/VTQR_ECOFEDUTs_c/OPD  TreatAsAtomicUnit=on
  VTQR_SPORTREDURateLimitDec_Nm : Outport
  wires:
  If/6 -> OPD/Action
  If/5 -> LV5/Action
  If/4 -> LV4/Action
  If/3 -> LV3/Action
  If/2 -> LV2/Action
  If/1 -> LV1/Action
  Invalid/1(VTQR_SL1REDUTqDecSR_Nm) -> Merge/7
  If/7 -> Invalid/Action
  [VTQD_TqTargetShaftSpd_rpm] -> Invalid/2(VTQD_TqTargetShaftSpd_rpm)
  [VTQR_REDUWhlTqReqSmoothDelay_Nm] -> Invalid/1(VTQR_REDUWhlTqReqSmoothDelay_Nm)
  VTQD_RegenMode_enum/1 -> [VTQD_RegenMode_enum]
  VTQD_TqTargetShaftSpd_rpm/1 -> [VTQD_TqTargetShaftSpd_rpm]
  VTQR_REDUWhlTqReqSmoothDelay_Nm/1 -> [VTQR_REDUWhlTqReqSmoothDelay_Nm]
  Merge/1 -> VTQR_SPORTREDURateLimitDec_Nm/1  "VTQR_SPORTREDURateLimitDec_Nm"
  Constant2/1 -> Equal2/2
  [VTQR_REDUWhlTqReqSmoothDelay_Nm] -> LV1/1(VTQR_REDUWhlTqReqSmoothDelay_Nm)
  [VTQD_TqTargetShaftSpd_rpm] -> LV3/2(VTQD_TqTargetShaftSpd_rpm)
  LV4/1(VTQR_SL4REDUTqDecSR_Nm) -> Merge/4
  Equal3/1 -> If/4
  [VTQD_RegenMode_enum] -> Equal1/1
  LV5/1(VTQR_SL5REDUTqIDecSR_Nm) -> Merge/5
  LV3/1(VTQR_SL3REDUTqDecSR_Nm) -> Merge/3
  [VTQD_RegenMode_enum] -> Equal3/1
  Equal1/1 -> If/2
  Equal4/1 -> If/5
  [VTQD_RegenMode_enum] -> Equal/1
  LV1/1(VTQR_SL1REDUTqDecSR_Nm) -> Merge/1
  Constant1/1 -> Equal1/2
  Equal/1 -> If/1
  [VTQD_TqTargetShaftSpd_rpm] -> LV5/2(VTQD_TqTargetShaftSpd_rpm)
  [VTQR_REDUWhlTqReqSmoothDelay_Nm] -> LV4/1(VTQR_REDUWhlTqReqSmoothDelay_Nm)
  Constant5/1 -> Equal5/2
  [VTQR_REDUWhlTqReqSmoothDelay_Nm] -> LV3/1(VTQR_REDUWhlTqReqSmoothDelay_Nm)
  [VTQD_TqTargetShaftSpd_rpm] -> LV4/2(VTQD_TqTargetShaftSpd_rpm)
  [VTQD_TqTargetShaftSpd_rpm] -> OPD/2(VTQD_TqTargetShaftSpd_rpm)
  [VTQR_REDUWhlTqReqSmoothDelay_Nm] -> LV5/1(VTQR_REDUWhlTqReqSmoothDelay_Nm)
  [VTQD_TqTargetShaftSpd_rpm] -> LV1/2(VTQD_TqTargetShaftSpd_rpm)
  [VTQD_RegenMode_enum] -> Equal2/1
  [VTQR_REDUWhlTqReqSmoothDelay_Nm] -> OPD/1(VTQR_REDUWhlTqReqSmoothDelay_Nm)
  [VTQD_RegenMode_enum] -> Equal5/1
  LV2/1(VTQR_SL2REDUTqDecSR_Nm) -> Merge/2
  [VTQR_REDUWhlTqReqSmoothDelay_Nm] -> LV2/1(VTQR_REDUWhlTqReqSmoothDelay_Nm)
  [VTQD_RegenMode_enum] -> Equal4/1
  OPD/1(VTQR_SOPDREDUTqDecSR_Nm) -> Merge/6
  Equal5/1 -> If/6
  Constant/1 -> Equal/2
  Constant4/1 -> Equal4/2
  Equal2/1 -> If/3
  Constant3/1 -> Equal3/2
  [VTQD_TqTargetShaftSpd_rpm] -> LV2/2(VTQD_TqTargetShaftSpd_rpm)

== system tqr/TQR/Determine Torque Request/TorqueArbitrament/TorqueSmooth/Rear wheel rate limit determination/VTQR_SPORTREDURateLimitInc_Nm ==
  VDHP_ActAPSPosn_pct : Inport
  VTQD_TqTargetShaftSpd_rpm : Inport  Port=2
  VTQD_RegenMode_enum : Inport  Port=3
  VTQR_REDUWhlTqReqSmoothDelay_Nm : Inport  Port=4
  Action Port : ActionPort
  Constant : Constant  Value=ENUM_REGENLEVEL_LV1
  Constant1 : Constant  Value=ENUM_REGENLEVEL_LV2
  Constant2 : Constant  Value=ENUM_REGENLEVEL_LV3
  Constant3 : Constant  Value=ENUM_REGENLEVEL_LV4
  Constant4 : Constant  Value=ENUM_REGENLEVEL_LV5
  Constant5 : Constant  Value=ENUM_REGENLEVEL_OPD
  Constant6 : Constant  Value=KTQR_EnSportRrIncGain_enum
  Constant7 : Constant  Value=ONE_FLOAT
  Equal{,1..5} (6 alike) : RelationalOperator  Operator===  OutDataTypeStr=boolean  RndMeth=Simplest
  If : If  NumInputs=6  IfExpression=u1~= 0  ElseIfExpressions=u2 ~= 0, u3 ~= 0,u4 ~= 0,u5~=0,u6~=0
  Invalid : Subsystem  TreatAsAtomicUnit=on
  LV1 : Subsystem  TreatAsAtomicUnit=on
  LV2 : Subsystem  TreatAsAtomicUnit=on
  LV3 : Subsystem  TreatAsAtomicUnit=on
  LV4 : Subsystem  TreatAsAtomicUnit=on
  LV5 : Subsystem  TreatAsAtomicUnit=on
  MTQR_Sport2TqRrIncGain_Z_c : Lookup_n-D  BreakpointsForDimension1=ATQR_Sport2TqRrIncGain_Y_pct  BreakpointsForDimension2=ATQR_Sport2TqRrIncGain_X_Nm  Table=MTQR_Sport2TqRrIncGain_Z_c  ExtrapMethod=Clip  InternalRulePriority=Speed  RndMeth=Simplest  InputSameDT=on
      settings: InputPortMap=u0,u1
  MTQR_Sport3TqRrIncGain_Z_c : Lookup_n-D  BreakpointsForDimension1=ATQR_Sport2TqRrIncGain_Y_pct  BreakpointsForDimension2=ATQR_Sport2TqRrIncGain_X_Nm  Table=MTQR_Sport3TqRrIncGain_Z_c  ExtrapMethod=Clip  InternalRulePriority=Speed  RndMeth=Simplest  InputSameDT=on
      settings: InputPortMap=u0,u1
  MTQR_Sport4TqRrIncGain_Z_c : Lookup_n-D  BreakpointsForDimension1=ATQR_Sport2TqRrIncGain_Y_pct  BreakpointsForDimension2=ATQR_Sport2TqRrIncGain_X_Nm  Table=MTQR_Sport4TqRrIncGain_Z_c  ExtrapMethod=Clip  InternalRulePriority=Speed  RndMeth=Simplest  InputSameDT=on
      settings: InputPortMap=u0,u1
  MTQR_Sport5TqRrIncGain_Z_c : Lookup_n-D  BreakpointsForDimension1=ATQR_Sport2TqRrIncGain_Y_pct  BreakpointsForDimension2=ATQR_Sport2TqRrIncGain_X_Nm  Table=MTQR_Sport5TqRrIncGain_Z_c  ExtrapMethod=Clip  InternalRulePriority=Speed  RndMeth=Simplest  InputSameDT=on
      settings: InputPortMap=u0,u1
  MTQR_SportOPDTqRrIncGain_Z_c : Lookup_n-D  BreakpointsForDimension1=ATQR_Sport2TqRrIncGain_Y_pct  BreakpointsForDimension2=ATQR_Sport2TqRrIncGain_X_Nm  Table=MTQR_SportOPDTqRrIncGain_Z_c  ExtrapMethod=Clip  InternalRulePriority=Speed  RndMeth=Simplest  InputSameDT=on
      settings: InputPortMap=u0,u1
  MTQR_SportTqRrIncGain_Z_c : Lookup_n-D  BreakpointsForDimension1=ATQR_SportTqRrIncGain_Y_pct  BreakpointsForDimension2=ATQR_SportTqRrIncGain_X_Nm  Table=MTQR_SportTqRrIncGain_Z_c  ExtrapMethod=Clip  InternalRulePriority=Speed  RndMeth=Simplest  InputSameDT=on
      settings: InputPortMap=u0,u1
  Merge : Merge  Inputs=7
  OPD : Subsystem  TreatAsAtomicUnit=on
  Relational Operator : RelationalOperator  OutDataTypeStr=boolean  RndMeth=Simplest
  Switch : Switch  Criteria=u2 > Threshold
  VTQR_SPORTREDURateLimitInc_Nm : Outport
  wires:
  If/7 -> Invalid/Action
  If/6 -> OPD/Action
  [VTQR_SportOPDTqRrIncGain_c] -> OPD/4(VTQR_SportOPDTqRrIncGain_c)
  [VTQR_Sport5TqRrIncGain_c] -> LV5/4(VTQR_Sport5TqRrIncGain_c)
  If/5 -> LV5/Action
  If/4 -> LV4/Action
  [VTQR_Sport4TqRrIncGain_c] -> LV4/4(VTQR_Sport4TqRrIncGain_c)
  If/3 -> LV3/Action
  [VTQR_Sport3TqRrIncGain_c] -> LV3/4(VTQR_Sport3TqRrIncGain_c)
  [VTQR_Sport2TqRrIncGain_c] -> LV2/4(VTQR_Sport2TqRrIncGain_c)
  If/2 -> LV2/Action
  If/1 -> LV1/Action
  [VTQR_REDUWhlTqReqSmoothDelay_Nm] -> MTQR_SportOPDTqRrIncGain_Z_c/2
  [VDHP_ActAPSPosn_pct] -> MTQR_SportOPDTqRrIncGain_Z_c/1
  [VDHP_ActAPSPosn_pct] -> MTQR_Sport5TqRrIncGain_Z_c/1
  [VTQR_REDUWhlTqReqSmoothDelay_Nm] -> MTQR_Sport5TqRrIncGain_Z_c/2
  [VTQR_REDUWhlTqReqSmoothDelay_Nm] -> MTQR_Sport4TqRrIncGain_Z_c/2
  [VDHP_ActAPSPosn_pct] -> MTQR_Sport4TqRrIncGain_Z_c/1
  [VDHP_ActAPSPosn_pct] -> MTQR_Sport3TqRrIncGain_Z_c/1
  [VTQR_REDUWhlTqReqSmoothDelay_Nm] -> MTQR_Sport3TqRrIncGain_Z_c/2
  [VTQR_REDUWhlTqReqSmoothDelay_Nm] -> MTQR_Sport2TqRrIncGain_Z_c/2
  [VDHP_ActAPSPosn_pct] -> MTQR_Sport2TqRrIncGain_Z_c/1
  MTQR_SportOPDTqRrIncGain_Z_c/1 -> [VTQR_SportOPDTqRrIncGain_c]  "VTQR_SportOPDTqRrIncGain_c"
  MTQR_Sport2TqRrIncGain_Z_c/1 -> [VTQR_Sport2TqRrIncGain_c]  "VTQR_Sport2TqRrIncGain_c"
  MTQR_Sport5TqRrIncGain_Z_c/1 -> [VTQR_Sport5TqRrIncGain_c]  "VTQR_Sport5TqRrIncGain_c"
  MTQR_Sport3TqRrIncGain_Z_c/1 -> [VTQR_Sport3TqRrIncGain_c]  "VTQR_Sport3TqRrIncGain_c"
  MTQR_Sport4TqRrIncGain_Z_c/1 -> [VTQR_Sport4TqRrIncGain_c]  "VTQR_Sport4TqRrIncGain_c"
  Switch/1 -> [VTQR_SportTqRrIncGain_c]  "VTQR_SportTqRrIncGain_c"
  [VTQD_RegenMode_enum] -> Relational Operator/1
  Relational Operator/1 -> Switch/2
  Constant7/1 -> Switch/3
  Constant6/1 -> Relational Operator/2
  MTQR_SportTqRrIncGain_Z_c/1 -> Switch/1
  [VTQR_SportTqRrIncGain_c] -> OPD/3(VTQR_SportTqRrIncGain_c)
  [VTQR_SportTqRrIncGain_c] -> LV5/3(VTQR_SportTqRrIncGain_c)
  [VTQR_SportTqRrIncGain_c] -> LV4/3(VTQR_SportTqRrIncGain_c)
  [VTQR_SportTqRrIncGain_c] -> LV3/3(VTQR_SportTqRrIncGain_c)
  [VTQR_SportTqRrIncGain_c] -> LV2/3(VTQR_SportTqRrIncGain_c)
  [VTQR_SportTqRrIncGain_c] -> LV1/3(VTQR_SportTqRrIncGain_c)
  VTQR_REDUWhlTqReqSmoothDelay_Nm/1 -> [VTQR_REDUWhlTqReqSmoothDelay_Nm]
  [VDHP_ActAPSPosn_pct] -> MTQR_SportTqRrIncGain_Z_c/1
  [VTQR_REDUWhlTqReqSmoothDelay_Nm] -> MTQR_SportTqRrIncGain_Z_c/2
  Invalid/1(VTQR_SL1REDUTqIncSR_Nm) -> Merge/7
  [VTQD_TqTargetShaftSpd_rpm] -> Invalid/2(VTQD_TqTargetShaftSpd_rpm)
  [VDHP_ActAPSPosn_pct] -> Invalid/1(VDHP_ActAPSPosn_pct)
  VTQD_RegenMode_enum/1 -> [VTQD_RegenMode_enum]
  [VTQD_TqTargetShaftSpd_rpm] -> LV4/2(VTQD_TqTargetShaftSpd_rpm)
  [VTQD_RegenMode_enum] -> Equal/1
  Equal/1 -> If/1
  Constant1/1 -> Equal1/2
  Equal4/1 -> If/5
  [VTQD_TqTargetShaftSpd_rpm] -> LV3/2(VTQD_TqTargetShaftSpd_rpm)
  Constant5/1 -> Equal5/2
  LV5/1(VTQR_SL5REDUTqIncSR_Nm) -> Merge/5
  [VTQD_RegenMode_enum] -> Equal5/1
  [VDHP_ActAPSPosn_pct] -> LV4/1(VDHP_ActAPSPosn_pct)
  LV3/1(VTQR_SL3REDUTqIncSR_Nm) -> Merge/3
  [VTQD_RegenMode_enum] -> Equal1/1
  LV4/1(VTQR_SL4REDUTqIncSR_Nm) -> Merge/4
  LV1/1(VTQR_SL1REDUTqIncSR_Nm) -> Merge/1
  VTQD_TqTargetShaftSpd_rpm/1 -> [VTQD_TqTargetShaftSpd_rpm]
  [VTQD_RegenMode_enum] -> Equal4/1
  Constant2/1 -> Equal2/2
  VDHP_ActAPSPosn_pct/1 -> [VDHP_ActAPSPosn_pct]
  Equal2/1 -> If/3
  Equal3/1 -> If/4
  Equal5/1 -> If/6
  [VDHP_ActAPSPosn_pct] -> OPD/1(VDHP_ActAPSPosn_pct)
  [VTQD_TqTargetShaftSpd_rpm] -> LV5/2(VTQD_TqTargetShaftSpd_rpm)
  [VDHP_ActAPSPosn_pct] -> LV1/1(VDHP_ActAPSPosn_pct)
  [VTQD_TqTargetShaftSpd_rpm] -> LV1/2(VTQD_TqTargetShaftSpd_rpm)
  LV2/1(VTQR_SL2REDUTqIncSR_Nm) -> Merge/2
  Constant4/1 -> Equal4/2
  Equal1/1 -> If/2
  [VTQD_RegenMode_enum] -> Equal3/1
  [VTQD_TqTargetShaftSpd_rpm] -> LV2/2(VTQD_TqTargetShaftSpd_rpm)
  [VDHP_ActAPSPosn_pct] -> LV3/1(VDHP_ActAPSPosn_pct)
  OPD/1(VTQR_SOPDREDUTqIncSR_Nm) -> Merge/6
  Constant/1 -> Equal/2
  Merge/1 -> VTQR_SPORTREDURateLimitInc_Nm/1  "VTQR_SPORTREDURateLimitInc_Nm"
  [VTQD_TqTargetShaftSpd_rpm] -> OPD/2(VTQD_TqTargetShaftSpd_rpm)
  [VDHP_ActAPSPosn_pct] -> LV5/1(VDHP_ActAPSPosn_pct)
  [VDHP_ActAPSPosn_pct] -> LV2/1(VDHP_ActAPSPosn_pct)
  Constant3/1 -> Equal3/2
  [VTQD_RegenMode_enum] -> Equal2/1

== system tqr/TQR/Determine Torque Request/TorqueArbitrament/TorqueSmooth/Rear wheel rate limit determination/VTQR_TCSREDURateLimitDec_Nm ==
  VTQR_REDUWhlTqReqSmoothDelay_Nm : Inport
  VTQD_TqTargetShaftSpd_rpm : Inport  Port=2
  Action Port : ActionPort
  MTQR_TCSREDUTqDecSR_Z_Nm : Lookup_n-D  BreakpointsForDimension1=ATQR_NL1REDUTqDecSR_Y_Nm  BreakpointsForDimension2=ATQR_NL1FEDUTqIncSR_X_rpm  Table=MTQR_TCSREDUTqDecSR_Z_Nm  InternalRulePriority=Speed  RndMeth=Simplest  InputSameDT=on
      settings: InputPortMap=u0,u1
  VTQR_TCSREDURateLimitDec_Nm : Outport
  wires:
  VTQD_TqTargetShaftSpd_rpm/1 -> MTQR_TCSREDUTqDecSR_Z_Nm/2
  VTQR_REDUWhlTqReqSmoothDelay_Nm/1 -> MTQR_TCSREDUTqDecSR_Z_Nm/1
  MTQR_TCSREDUTqDecSR_Z_Nm/1 -> VTQR_TCSREDURateLimitDec_Nm/1

== system tqr/TQR/Determine Torque Request/TorqueArbitrament/TorqueSmooth/Rear wheel rate limit determination/VTQR_TCSREDURateLimitInc_Nm ==
  VDHP_ActAPSPosn_pct : Inport
  VTQD_TqTargetShaftSpd_rpm : Inport  Port=2
  Action Port : ActionPort
  MTQR_TCSREDUTqIncSR_Z_Nm : Lookup_n-D  BreakpointsForDimension1=ATQR_NL1FEDUTqIncSR_Y_pct  BreakpointsForDimension2=ATQR_NL1FEDUTqIncSR_X_rpm  Table=MTQR_TCSREDUTqIncSR_Z_Nm  InternalRulePriority=Speed  RndMeth=Simplest  InputSameDT=on
      settings: InputPortMap=u0,u1
  VTQR_TCSREDURateLimitInc_Nm : Outport
  wires:
  MTQR_TCSREDUTqIncSR_Z_Nm/1 -> VTQR_TCSREDURateLimitInc_Nm/1
  VTQD_TqTargetShaftSpd_rpm/1 -> MTQR_TCSREDUTqIncSR_Z_Nm/2
  VDHP_ActAPSPosn_pct/1 -> MTQR_TCSREDUTqIncSR_Z_Nm/1

== system tqr/TQR/Determine Torque Request/TorqueArbitrament/TorqueSmooth/Front First order filter input tau map and determination/VTQR_ECOFEDUTs_c/Invalid ==
  VTQR_FEDUWhlTqReqSmoothDelay_Nm : Inport
  VTQD_TqTargetShaftSpd_rpm : Inport  Port=2
  VTQD_RollRegenEnable_flg : Inport  Port=3
  Action Port : ActionPort
  MTQR_EL1FEDUTs_Z_c : Lookup_n-D  BreakpointsForDimension1=ATQR_EL1FEDUTs_Y_Nm  BreakpointsForDimension2=ATQR_EL1FEDUTs_X_rpm  Table=MTQR_EL1FEDUTs_Z_c  ExtrapMethod=Clip  InternalRulePriority=Speed  RndMeth=Simplest  InputSameDT=on
      settings: InputPortMap=u0,u1
  MTQR_FEDUEL1RegenTs_Y_c : Lookup_n-D  NumberOfTableDimensions=1  BreakpointsForDimension1=ATQR_FEDUEL1RegenTs_X_rpm  BreakpointsForDimension2=ATQR_EL1FEDUTs_X_rpm  Table=MTQR_FEDUEL1RegenTs_Y_c  ExtrapMethod=Clip  InternalRulePriority=Speed  RndMeth=Simplest  InputSameDT=on
  Switch : Switch  Criteria=u2 ~= 0
  VTQR_EL1FEDUTsOrRegen_C : Outport
  wires:
  VTQD_RollRegenEnable_flg/1 -> Switch/2
  VTQR_FEDUWhlTqReqSmoothDelay_Nm/1 -> [VTQR_FEDUWhlTqReqSmoothDelay_Nm]
  VTQD_TqTargetShaftSpd_rpm/1 -> [VTQD_TqTargetShaftSpd_rpm]
  [VTQR_FEDUWhlTqReqSmoothDelay_Nm] -> MTQR_EL1FEDUTs_Z_c/1
  Switch/1 -> VTQR_EL1FEDUTsOrRegen_C/1
  MTQR_EL1FEDUTs_Z_c/1 -> Switch/3
  MTQR_FEDUEL1RegenTs_Y_c/1 -> Switch/1
  [VTQD_TqTargetShaftSpd_rpm] -> MTQR_FEDUEL1RegenTs_Y_c/1
  [VTQD_TqTargetShaftSpd_rpm] -> MTQR_EL1FEDUTs_Z_c/2

== system tqr/TQR/Determine Torque Request/TorqueArbitrament/TorqueSmooth/Front First order filter input tau map and determination/VTQR_ECOFEDUTs_c/LV1 ==
  VTQR_FEDUWhlTqReqSmoothDelay_Nm : Inport
  VTQD_TqTargetShaftSpd_rpm : Inport  Port=2
  VTQD_RollRegenEnable_flg : Inport  Port=3
  Action Port : ActionPort
  MTQR_EL1FEDUTs_Z_c : Lookup_n-D  BreakpointsForDimension1=ATQR_EL1FEDUTs_Y_Nm  BreakpointsForDimension2=ATQR_EL1FEDUTs_X_rpm  Table=MTQR_EL1FEDUTs_Z_c  ExtrapMethod=Clip  InternalRulePriority=Speed  RndMeth=Simplest  InputSameDT=on
      settings: InputPortMap=u0,u1
  MTQR_FEDUEL1RegenTs_Y_c : Lookup_n-D  NumberOfTableDimensions=1  BreakpointsForDimension1=ATQR_FEDUEL1RegenTs_X_rpm  BreakpointsForDimension2=ATQR_EL1FEDUTs_X_rpm  Table=MTQR_FEDUEL1RegenTs_Y_c  ExtrapMethod=Clip  InternalRulePriority=Speed  RndMeth=Simplest  InputSameDT=on
  Switch : Switch  Criteria=u2 ~= 0
  VTQR_EL1FEDUTsOrRegen_C : Outport
  wires:
  [VTQD_TqTargetShaftSpd_rpm] -> MTQR_EL1FEDUTs_Z_c/2
  [VTQD_TqTargetShaftSpd_rpm] -> MTQR_FEDUEL1RegenTs_Y_c/1
  MTQR_FEDUEL1RegenTs_Y_c/1 -> Switch/1
  MTQR_EL1FEDUTs_Z_c/1 -> Switch/3
  Switch/1 -> VTQR_EL1FEDUTsOrRegen_C/1
  [VTQR_FEDUWhlTqReqSmoothDelay_Nm] -> MTQR_EL1FEDUTs_Z_c/1
  VTQD_TqTargetShaftSpd_rpm/1 -> [VTQD_TqTargetShaftSpd_rpm]
  VTQR_FEDUWhlTqReqSmoothDelay_Nm/1 -> [VTQR_FEDUWhlTqReqSmoothDelay_Nm]
  VTQD_RollRegenEnable_flg/1 -> Switch/2

== system tqr/TQR/Determine Torque Request/TorqueArbitrament/TorqueSmooth/Front First order filter input tau map and determination/VTQR_ECOFEDUTs_c/LV2 ==
  VTQR_FEDUWhlTqReqSmoothDelay_Nm : Inport
  VTQD_TqTargetShaftSpd_rpm : Inport  Port=2
  Action Port : ActionPort
  MTQR_EL2FEDUTs_Z_c : Lookup_n-D  BreakpointsForDimension1=ATQR_EL1FEDUTs_Y_Nm  BreakpointsForDimension2=ATQR_EL1FEDUTs_X_rpm  Table=MTQR_EL2FEDUTs_Z_c  ExtrapMethod=Clip  InternalRulePriority=Speed  RndMeth=Simplest  InputSameDT=on
      settings: InputPortMap=u0,u1
  VTQR_EL2FEDUTs_c : Outport
  wires:
  MTQR_EL2FEDUTs_Z_c/1 -> VTQR_EL2FEDUTs_c/1
  VTQD_TqTargetShaftSpd_rpm/1 -> MTQR_EL2FEDUTs_Z_c/2
  VTQR_FEDUWhlTqReqSmoothDelay_Nm/1 -> MTQR_EL2FEDUTs_Z_c/1

== system tqr/TQR/Determine Torque Request/TorqueArbitrament/TorqueSmooth/Front First order filter input tau map and determination/VTQR_ECOFEDUTs_c/LV3 ==
  VTQR_FEDUWhlTqReqSmoothDelay_Nm : Inport
  VTQD_TqTargetShaftSpd_rpm : Inport  Port=2
  Action Port : ActionPort
  MTQR_EL3FEDUTs_Z_c : Lookup_n-D  BreakpointsForDimension1=ATQR_EL1FEDUTs_Y_Nm  BreakpointsForDimension2=ATQR_EL1FEDUTs_X_rpm  Table=MTQR_EL3FEDUTs_Z_c  ExtrapMethod=Clip  InternalRulePriority=Speed  RndMeth=Simplest  InputSameDT=on
      settings: InputPortMap=u0,u1
  VTQR_EL3FEDUTs_c : Outport
  wires:
  MTQR_EL3FEDUTs_Z_c/1 -> VTQR_EL3FEDUTs_c/1
  VTQD_TqTargetShaftSpd_rpm/1 -> MTQR_EL3FEDUTs_Z_c/2
  VTQR_FEDUWhlTqReqSmoothDelay_Nm/1 -> MTQR_EL3FEDUTs_Z_c/1

== system tqr/TQR/Determine Torque Request/TorqueArbitrament/TorqueSmooth/Front First order filter input tau map and determination/VTQR_ECOFEDUTs_c/LV4 ==
  VTQR_FEDUWhlTqReqSmoothDelay_Nm : Inport
  VTQD_TqTargetShaftSpd_rpm : Inport  Port=2
  Action Port : ActionPort
  MTQR_EL4FEDUTs_Z_c : Lookup_n-D  BreakpointsForDimension1=ATQR_EL1FEDUTs_Y_Nm  BreakpointsForDimension2=ATQR_EL1FEDUTs_X_rpm  Table=MTQR_EL4FEDUTs_Z_c  ExtrapMethod=Clip  InternalRulePriority=Speed  RndMeth=Simplest  InputSameDT=on
      settings: InputPortMap=u0,u1
  VTQR_EL4FEDUTs_c : Outport
  wires:
  MTQR_EL4FEDUTs_Z_c/1 -> VTQR_EL4FEDUTs_c/1
  VTQD_TqTargetShaftSpd_rpm/1 -> MTQR_EL4FEDUTs_Z_c/2
  VTQR_FEDUWhlTqReqSmoothDelay_Nm/1 -> MTQR_EL4FEDUTs_Z_c/1

== system tqr/TQR/Determine Torque Request/TorqueArbitrament/TorqueSmooth/Front First order filter input tau map and determination/VTQR_ECOFEDUTs_c/LV5 ==
  VTQR_FEDUWhlTqReqSmoothDelay_Nm : Inport
  VTQD_TqTargetShaftSpd_rpm : Inport  Port=2
  Action Port : ActionPort
  MTQR_EL5FEDUTs_Z_c : Lookup_n-D  BreakpointsForDimension1=ATQR_EL1FEDUTs_Y_Nm  BreakpointsForDimension2=ATQR_EL1FEDUTs_X_rpm  Table=MTQR_EL5FEDUTs_Z_c  ExtrapMethod=Clip  InternalRulePriority=Speed  RndMeth=Simplest  InputSameDT=on
      settings: InputPortMap=u0,u1
  VTQR_EL5FEDUTs_c : Outport
  wires:
  MTQR_EL5FEDUTs_Z_c/1 -> VTQR_EL5FEDUTs_c/1
  VTQD_TqTargetShaftSpd_rpm/1 -> MTQR_EL5FEDUTs_Z_c/2
  VTQR_FEDUWhlTqReqSmoothDelay_Nm/1 -> MTQR_EL5FEDUTs_Z_c/1

== system tqr/TQR/Determine Torque Request/TorqueArbitrament/TorqueSmooth/Front First order filter input tau map and determination/VTQR_ECOFEDUTs_c/OPD ==
  VTQR_FEDUWhlTqReqSmoothDelay_Nm : Inport
  VTQD_TqTargetShaftSpd_rpm : Inport  Port=2
  Action Port : ActionPort
  MTQR_EOPDFEDUTs_Z_c : Lookup_n-D  BreakpointsForDimension1=ATQR_EL1FEDUTs_Y_Nm  BreakpointsForDimension2=ATQR_EL1FEDUTs_X_rpm  Table=MTQR_EOPDFEDUTs_Z_c  ExtrapMethod=Clip  InternalRulePriority=Speed  RndMeth=Simplest  InputSameDT=on
      settings: InputPortMap=u0,u1
  VTQR_EOPDFEDUTs_c : Outport
  wires:
  MTQR_EOPDFEDUTs_Z_c/1 -> VTQR_EOPDFEDUTs_c/1
  VTQD_TqTargetShaftSpd_rpm/1 -> MTQR_EOPDFEDUTs_Z_c/2
  VTQR_FEDUWhlTqReqSmoothDelay_Nm/1 -> MTQR_EOPDFEDUTs_Z_c/1

== system tqr/TQR/Determine Torque Request/TorqueArbitrament/TorqueSmooth/Front First order filter input tau map and determination/VTQR_NORMALFEDUTs_c/Invalid ==
  VTQR_FEDUWhlTqReqSmoothDelay_Nm : Inport
  VTQD_TqTargetShaftSpd_rpm : Inport  Port=2
  Action Port : ActionPort
  MTQR_NL1FEDUTs_Z_c : Lookup_n-D  BreakpointsForDimension1=ATQR_NL1FEDUTs_Y_Nm  BreakpointsForDimension2=ATQR_NL1FEDUTs_X_rpm  Table=MTQR_NL1FEDUTs_Z_c  ExtrapMethod=Clip  InternalRulePriority=Speed  RndMeth=Simplest  InputSameDT=on
      settings: InputPortMap=u0,u1
  VTQR_NL1FEDUTs_c : Outport
  wires:
  MTQR_NL1FEDUTs_Z_c/1 -> VTQR_NL1FEDUTs_c/1
  VTQD_TqTargetShaftSpd_rpm/1 -> MTQR_NL1FEDUTs_Z_c/2
  VTQR_FEDUWhlTqReqSmoothDelay_Nm/1 -> MTQR_NL1FEDUTs_Z_c/1

== system tqr/TQR/Determine Torque Request/TorqueArbitrament/TorqueSmooth/Front First order filter input tau map and determination/VTQR_NORMALFEDUTs_c/LV1 ==
  VTQR_FEDUWhlTqReqSmoothDelay_Nm : Inport
  VTQD_TqTargetShaftSpd_rpm : Inport  Port=2
  Action Port : ActionPort
  MTQR_NL1FEDUTs_Z_c : Lookup_n-D  BreakpointsForDimension1=ATQR_NL1FEDUTs_Y_Nm  BreakpointsForDimension2=ATQR_NL1FEDUTs_X_rpm  Table=MTQR_NL1FEDUTs_Z_c  ExtrapMethod=Clip  InternalRulePriority=Speed  RndMeth=Simplest  InputSameDT=on
      settings: InputPortMap=u0,u1
  VTQR_NL1FEDUTs_c : Outport
  wires:
  VTQR_FEDUWhlTqReqSmoothDelay_Nm/1 -> MTQR_NL1FEDUTs_Z_c/1
  VTQD_TqTargetShaftSpd_rpm/1 -> MTQR_NL1FEDUTs_Z_c/2
  MTQR_NL1FEDUTs_Z_c/1 -> VTQR_NL1FEDUTs_c/1

== system tqr/TQR/Determine Torque Request/TorqueArbitrament/TorqueSmooth/Front First order filter input tau map and determination/VTQR_NORMALFEDUTs_c/LV2 ==
  VTQR_FEDUWhlTqReqSmoothDelay_Nm : Inport
  VTQD_TqTargetShaftSpd_rpm : Inport  Port=2
  Action Port : ActionPort
  MTQR_NL2FEDUTs_Z_c : Lookup_n-D  BreakpointsForDimension1=ATQR_NL1FEDUTs_Y_Nm  BreakpointsForDimension2=ATQR_NL1FEDUTs_X_rpm  Table=MTQR_NL2FEDUTs_Z_c  ExtrapMethod=Clip  InternalRulePriority=Speed  RndMeth=Simplest  InputSameDT=on
      settings: InputPortMap=u0,u1
  VTQR_NL2FEDUTs_c : Outport
  wires:
  MTQR_NL2FEDUTs_Z_c/1 -> VTQR_NL2FEDUTs_c/1
  VTQD_TqTargetShaftSpd_rpm/1 -> MTQR_NL2FEDUTs_Z_c/2
  VTQR_FEDUWhlTqReqSmoothDelay_Nm/1 -> MTQR_NL2FEDUTs_Z_c/1

== system tqr/TQR/Determine Torque Request/TorqueArbitrament/TorqueSmooth/Front First order filter input tau map and determination/VTQR_NORMALFEDUTs_c/LV3 ==
  VTQR_FEDUWhlTqReqSmoothDelay_Nm : Inport
  VTQD_TqTargetShaftSpd_rpm : Inport  Port=2
  Action Port : ActionPort
  MTQR_NL3FEDUTs_Z_c : Lookup_n-D  BreakpointsForDimension1=ATQR_NL1FEDUTs_Y_Nm  BreakpointsForDimension2=ATQR_NL1FEDUTs_X_rpm  Table=MTQR_NL3FEDUTs_Z_c  ExtrapMethod=Clip  InternalRulePriority=Speed  RndMeth=Simplest  InputSameDT=on
      settings: InputPortMap=u0,u1
  VTQR_NL3FEDUTs_c : Outport
  wires:
  MTQR_NL3FEDUTs_Z_c/1 -> VTQR_NL3FEDUTs_c/1
  VTQD_TqTargetShaftSpd_rpm/1 -> MTQR_NL3FEDUTs_Z_c/2
  VTQR_FEDUWhlTqReqSmoothDelay_Nm/1 -> MTQR_NL3FEDUTs_Z_c/1

== system tqr/TQR/Determine Torque Request/TorqueArbitrament/TorqueSmooth/Front First order filter input tau map and determination/VTQR_NORMALFEDUTs_c/LV4 ==
  VTQR_FEDUWhlTqReqSmoothDelay_Nm : Inport
  VTQD_TqTargetShaftSpd_rpm : Inport  Port=2
  Action Port : ActionPort
  MTQR_NL4FEDUTs_Z_c : Lookup_n-D  BreakpointsForDimension1=ATQR_NL1FEDUTs_Y_Nm  BreakpointsForDimension2=ATQR_NL1FEDUTs_X_rpm  Table=MTQR_NL4FEDUTs_Z_c  ExtrapMethod=Clip  InternalRulePriority=Speed  RndMeth=Simplest  InputSameDT=on
      settings: InputPortMap=u0,u1
  VTQR_NL4FEDUTs_c : Outport
  wires:
  MTQR_NL4FEDUTs_Z_c/1 -> VTQR_NL4FEDUTs_c/1
  VTQD_TqTargetShaftSpd_rpm/1 -> MTQR_NL4FEDUTs_Z_c/2
  VTQR_FEDUWhlTqReqSmoothDelay_Nm/1 -> MTQR_NL4FEDUTs_Z_c/1

== system tqr/TQR/Determine Torque Request/TorqueArbitrament/TorqueSmooth/Front First order filter input tau map and determination/VTQR_NORMALFEDUTs_c/LV5 ==
  VTQR_FEDUWhlTqReqSmoothDelay_Nm : Inport
  VTQD_TqTargetShaftSpd_rpm : Inport  Port=2
  Action Port : ActionPort
  MTQR_NL5FEDUTs_Z_c : Lookup_n-D  BreakpointsForDimension1=ATQR_NL1FEDUTs_Y_Nm  BreakpointsForDimension2=ATQR_NL1FEDUTs_X_rpm  Table=MTQR_NL5FEDUTs_Z_c  ExtrapMethod=Clip  InternalRulePriority=Speed  RndMeth=Simplest  InputSameDT=on
      settings: InputPortMap=u0,u1
  VTQR_NL5FEDUTs_c : Outport
  wires:
  MTQR_NL5FEDUTs_Z_c/1 -> VTQR_NL5FEDUTs_c/1
  VTQD_TqTargetShaftSpd_rpm/1 -> MTQR_NL5FEDUTs_Z_c/2
  VTQR_FEDUWhlTqReqSmoothDelay_Nm/1 -> MTQR_NL5FEDUTs_Z_c/1

== system tqr/TQR/Determine Torque Request/TorqueArbitrament/TorqueSmooth/Front First order filter input tau map and determination/VTQR_NORMALFEDUTs_c/OPD ==
  VTQR_FEDUWhlTqReqSmoothDelay_Nm : Inport
  VTQD_TqTargetShaftSpd_rpm : Inport  Port=2
  Action Port : ActionPort
  MTQR_NOPDFEDUTs_Z_c : Lookup_n-D  BreakpointsForDimension1=ATQR_NL1FEDUTs_Y_Nm  BreakpointsForDimension2=ATQR_NL1FEDUTs_X_rpm  Table=MTQR_NOPDFEDUTs_Z_c  ExtrapMethod=Clip  InternalRulePriority=Speed  RndMeth=Simplest  InputSameDT=on
      settings: InputPortMap=u0,u1
  VTQR_NOPDFEDUTs_c : Outport
  wires:
  MTQR_NOPDFEDUTs_Z_c/1 -> VTQR_NOPDFEDUTs_c/1
  VTQD_TqTargetShaftSpd_rpm/1 -> MTQR_NOPDFEDUTs_Z_c/2
  VTQR_FEDUWhlTqReqSmoothDelay_Nm/1 -> MTQR_NOPDFEDUTs_Z_c/1

== system tqr/TQR/Determine Torque Request/TorqueArbitrament/TorqueSmooth/Front First order filter input tau map and determination/VTQR_SPORTFEDUTs_c/Invalid ==
  VTQR_FEDUWhlTqReqSmoothDelay_Nm : Inport
  VTQD_TqTargetShaftSpd_rpm : Inport  Port=2
  Action Port : ActionPort
  MTQR_SL1FEDUTs_Z_c : Lookup_n-D  BreakpointsForDimension1=ATQR_SL1FEDUTs_Y_Nm  BreakpointsForDimension2=ATQR_SL1FEDUTs_X_rpm  Table=MTQR_SL1FEDUTs_Z_c  ExtrapMethod=Clip  InternalRulePriority=Speed  RndMeth=Simplest  InputSameDT=on
      settings: InputPortMap=u0,u1
  VTQR_SL1FEDUTs_c : Outport
  wires:
  MTQR_SL1FEDUTs_Z_c/1 -> VTQR_SL1FEDUTs_c/1
  VTQD_TqTargetShaftSpd_rpm/1 -> MTQR_SL1FEDUTs_Z_c/2
  VTQR_FEDUWhlTqReqSmoothDelay_Nm/1 -> MTQR_SL1FEDUTs_Z_c/1
